simulink model "pos_control2"  (R2016b)
settings: Solver=ode3  StartTime=0.0  StopTime=50  FixedStep=0.0025  RelTol=1e-3
model workspace: external: MATLAB File /home/zhouhua/Clobotics/px4_simulink/px4_motor_order/pos_control_px4_order/para_pos.m (data not in the file)
values from neighbouring files (symbols this model uses):
  Ang_Pos_initial = [x0, y0, z0, phi0, theta0, psi0]    [para_pos.m]
  b = (middle_cruise_speed - c) / a    [get_vel_close.m]    (also in gradual.m = y_low - a * x_low; para_pos.m = 1.38089806e-06)
  compensation_gain = 1    [para_pos.m]
  d = 4.152245751114358e-08    (= 4.15224575111e-08)    [para_pos.m]
  dt = 0.0025    [para_pos.m]
  g = 9.8    [para_pos.m]
  Ix = 0.676603    [para_pos.m]
  Iy = 0.996394    [para_pos.m]
  Iz = 0.640393    [para_pos.m]
  L = 0.6    [para_pos.m]
  m = 10.3551    [para_pos.m]
  omiga1 = 0000    (= 0)    [para_pos.m]
  omiga2 = 0000    (= 0)    [para_pos.m]
  omiga3 = 0000    (= 0)    [para_pos.m]
  omiga4 = 0000    (= 0)    [para_pos.m]
  thrust_rpyt_low = [0,0,0,0,0,0]    [para_pos.m]
  thrust_rpyt_up = [1,1,1,1,1,1]    [para_pos.m]
  X1_PWM_MotorVel = -0.0023    [para_pos.m]
  X2_PWM_MotorVel = 13.6492    [para_pos.m]
  X3_PWM_MotorVel = -1.2185e+4    (= -12185)    [para_pos.m]
undefined symbols (not defined in the file or in its folder): bool_pos, control_mode, def, par, par_input, par_pos, position_setpoint
libraries: simulink x1
(part 1 of 2)
settings Model: Creator=root  LastModifiedBy=zhouhua
settings OptimizationCC: DefaultParameterBehavior=Inlined
settings DebuggingCC: ParameterTunabilityLossMsg=error
settings HardwareCC: ProdBitPerLong=64  ProdHWDeviceType=Intel->x86-64 (Linux 64)
settings RTWCC: SystemTargetFile=ert.tlc  TemplateMakefile=ert_default_tmf  Description=Embedded Coder  GenerateReport=on  IncludeHyperlinkInReport=on  LaunchReport=on  GenerateTraceInfo=on  GenerateTraceReport=on  GenerateTraceReportSl=on  GenerateTraceReportSf=on  GenerateTraceReportEml=on
settings CodeAppCC: ForceParamTrailComments=on  IgnoreCustomStorageClasses=off  OperatorAnnotations=on  SimulinkDataObjDesc=on  SFDataObjDesc=on  MATLABFcnDesc=on  InsertBlockDesc=on  MATLABSourceComments=on
settings ERTTargetCC: TargetLangStandard=C99 (ISO)  GenerateSampleERTMain=on  InlinedParameterPlacement=NonHierarchical  ERTCustomFileTemplate=example_file_process.tlc

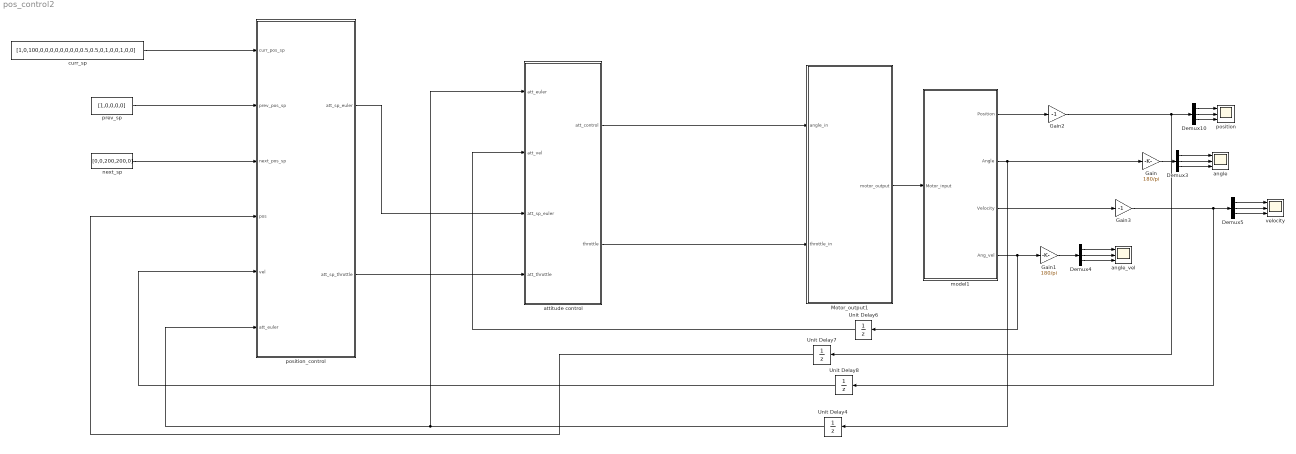
== system pos_control2 ==
  Demux{3..5,10} (4 alike) : Demux  Outputs=3
  Gain : Gain  Gain=180/pi
  Gain1 : Gain  Gain=180/pi
  Gain2 : Gain  Gain=-1
  Gain3 : Gain  Gain=-1
  Motor_output1 : Subsystem
  Unit Delay{4,6..8} (4 alike) : UnitDelay  InitialCondition=[0,0,0]  SampleTime=-1
  angle : Scope  NumInputPorts=3
  angle_vel : Scope  NumInputPorts=3
  attitude control : Subsystem
  curr_sp : Constant  Value=[1,0,100,0,0,0,0,0,0,0,0,0.5,0.5,0,1,0,0,1,0,0]
  model1 : Subsystem
  next_sp : Constant  Value=[0,0,200,200,0]
  position : Scope  NumInputPorts=3
  position_control : Subsystem
  prev_sp : Constant  Value=[1,0,0,0,0]
  velocity : Scope  NumInputPorts=3
  wires:
  Unit Delay4/1 -> position_control/6(att_euler), attitude control/1(att_euler)
  Unit Delay7/1 -> position_control/4(pos)
  Unit Delay8/1 -> position_control/5(vel)
  model1/2(Angle) -> Gain/1, Unit Delay4/1
  model1/4(Ang_vel) -> Gain1/1, Unit Delay6/1
  Gain2/1 -> Unit Delay7/1, Demux10/1
  model1/1(Position) -> Gain2/1
  Gain/1 -> Demux3/1
  Demux3/1 -> angle/1
  Demux3/2 -> angle/2
  Demux3/3 -> angle/3
  Demux4/1 -> angle_vel/1
  Demux4/2 -> angle_vel/2
  Demux4/3 -> angle_vel/3
  model1/3(Velocity) -> Gain3/1
  Demux5/1 -> velocity/1
  Demux5/2 -> velocity/2
  Demux5/3 -> velocity/3
  Gain1/1 -> Demux4/1
  Unit Delay6/1 -> attitude control/2(att_vel)
  Demux10/1 -> position/1
  Demux10/2 -> position/2
  Demux10/3 -> position/3
  Gain3/1 -> Demux5/1, Unit Delay8/1
  attitude control/1(att_control) -> Motor_output1/1(angle_in)
  attitude control/2(throttle) -> Motor_output1/2(throttle_in)
  position_control/1(att_sp_euler) -> attitude control/3(att_sp_euler)
  position_control/2(att_sp_throttle) -> attitude control/4(att_throttle)
  curr_sp/1 -> position_control/1(curr_pos_sp)
  prev_sp/1 -> position_control/2(prev_pos_sp)
  next_sp/1 -> position_control/3(next_pos_sp)
  Motor_output1/1(motor_output) -> model1/1(Motor_input)

== system pos_control2/Motor_output1 ==
  angle_in : Inport
  throttle_in : Inport  Port=2
  Display : Display
  output_armed_stabilizing : Subsystem
  output_to_motors : Subsystem
  motor_output : Outport
  wires:
  angle_in/1 -> Display/1, output_armed_stabilizing/1(In1)
  throttle_in/1 -> output_armed_stabilizing/2(In2)  "[0,1]"
  output_armed_stabilizing/1(thrust_rpyt_out) -> output_to_motors/1(thrust_in)
  output_to_motors/1(motor_ouput) -> motor_output/1

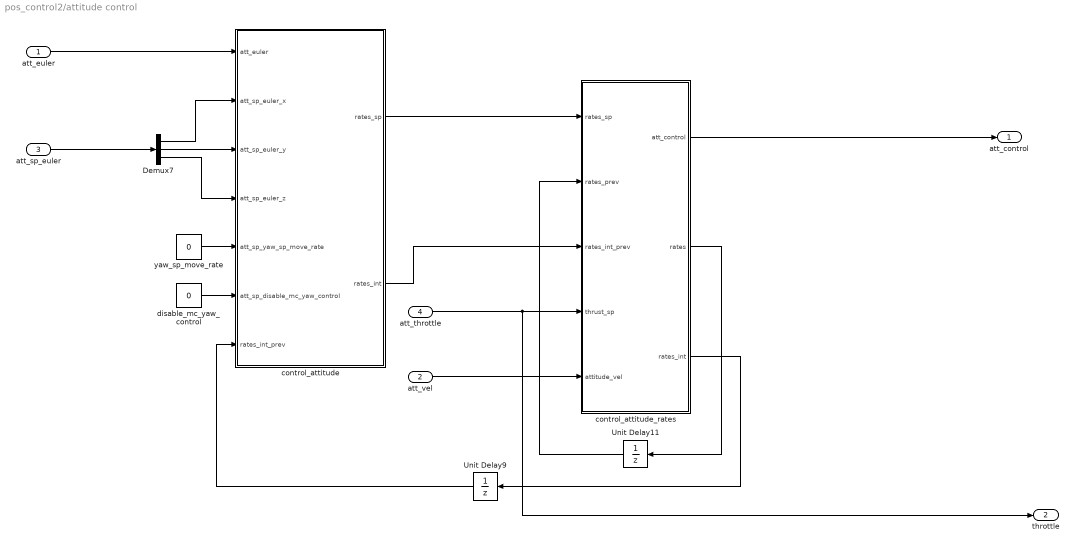
== system pos_control2/attitude control ==
  att_euler : Inport
  att_vel : Inport  Port=2
  att_sp_euler : Inport  Port=3
  att_throttle : Inport  Port=4
  Demux7 : Demux  Outputs=3
  Unit Delay11 : UnitDelay  InitialCondition=[0,0,0]  SampleTime=-1
  Unit Delay9 : UnitDelay  InitialCondition=[0,0,0]  SampleTime=-1
  control_attitude : MATLAB Function  TreatAsAtomicUnit=on
  control_attitude_rates : MATLAB Function  TreatAsAtomicUnit=on
  disable_mc_yaw_control : Constant  Value=0
  yaw_sp_move_rate : Constant  Value=0
  att_control : Outport
  throttle : Outport  Port=2
  wires:
  att_euler/1 -> control_attitude/1(att_euler)
  control_attitude_rates/3(rates_int) -> Unit Delay9/1
  control_attitude/2(rates_int) -> control_attitude_rates/3(rates_int_prev)
  control_attitude_rates/2(rates) -> Unit Delay11/1
  Unit Delay9/1 -> control_attitude/7(rates_int_prev)
  Unit Delay11/1 -> control_attitude_rates/2(rates_prev)
  yaw_sp_move_rate/1 -> control_attitude/5(att_sp_yaw_sp_move_rate)
  disable_mc_yaw_control/1 -> control_attitude/6(att_sp_disable_mc_yaw_control)
  control_attitude_rates/1(att_control) -> att_control/1
  control_attitude/1(rates_sp) -> control_attitude_rates/1(rates_sp)
  att_vel/1 -> control_attitude_rates/5(attitude_vel)
  Demux7/1 -> control_attitude/2(att_sp_euler_x)
  Demux7/2 -> control_attitude/3(att_sp_euler_y)
  Demux7/3 -> control_attitude/4(att_sp_euler_z)
  att_throttle/1 -> throttle/1, control_attitude_rates/4(thrust_sp)
  att_sp_euler/1 -> Demux7/1

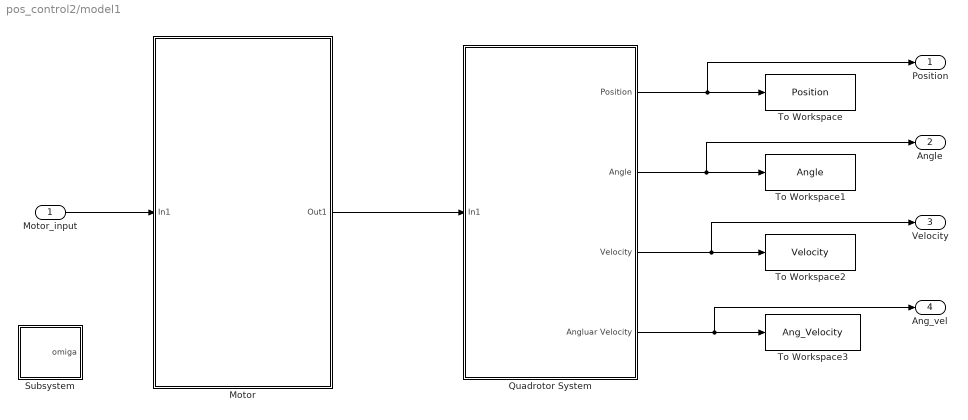
== system pos_control2/model1 ==
  Motor_input : Inport
  " Quadrotor System" : Subsystem
  Motor : Subsystem
  Subsystem : Subsystem
  To Workspace : ToWorkspace  VariableName=Position  SampleTime=-1
  To Workspace1 : ToWorkspace  VariableName=Angle  SampleTime=-1
  To Workspace2 : ToWorkspace  VariableName=Velocity  SampleTime=-1
  To Workspace3 : ToWorkspace  VariableName=Ang_Velocity  SampleTime=-1
  Position : Outport
  Angle : Outport  Port=2
  Velocity : Outport  Port=3
  Ang_vel : Outport  Port=4
  wires:
  Motor/1(Out1) -> " Quadrotor System"/1(In1)
  " Quadrotor System"/1(Position) -> Position/1, To Workspace/1
  " Quadrotor System"/3(Velocity) -> Velocity/1, To Workspace2/1
  " Quadrotor System"/4(Angluar Velocity) -> Ang_vel/1, To Workspace3/1
  Motor_input/1 -> Motor/1(In1)
  " Quadrotor System"/2(Angle) -> Angle/1, To Workspace1/1

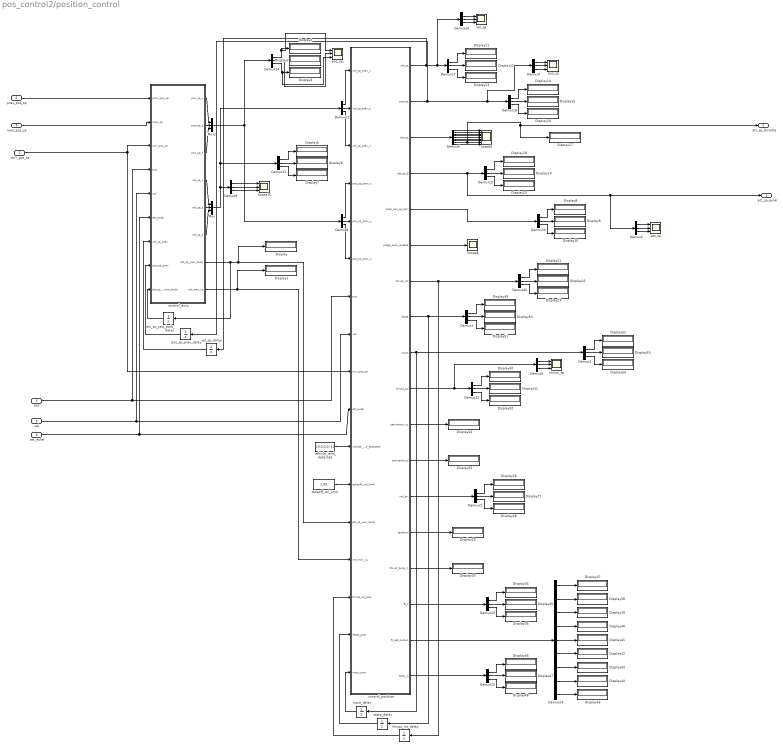
== system pos_control2/position_control ==
  curr_pos_sp : Inport
  prev_pos_sp : Inport  Port=2
  next_pos_sp : Inport  Port=3
  pos : Inport  Port=4
  vel : Inport  Port=5
  att_euler : Inport  Port=6
  Demux{1..5,8..10,12,14..23,25} (20 alike) : Demux  Outputs=3
  Demux24 : Demux  Outputs=9
  Demux6 : Demux  Outputs=9
  Display{,1..54} (55 alike) : Display
  Mux : Mux  Inputs=3
  Mux1 : Mux  Inputs=3
  Scope10 : Scope  NumInputPorts=3
  Scope5 : Scope  NumInputPorts=9
  Scope6 : Scope
  att_sp : Scope  NumInputPorts=3
  att_sp_yaw_body_delay : UnitDelay  InitialCondition=[0]  SampleTime=-1
  control_auto : MATLAB Function  TreatAsAtomicUnit=on
  control_position : MATLAB Function  TreatAsAtomicUnit=on
  input_delay : UnitDelay  InitialCondition=[0,0,0]  SampleTime=-1
  pos_sp : Scope  NumInputPorts=3
  "pos_sp_ " : Scope  NumInputPorts=3
  pos_sp_prev_delay : UnitDelay  InitialCondition=[0]  SampleTime=-1
  state_delay : UnitDelay  InitialCondition=[0,0,0]  SampleTime=-1
  takeoff_vel_limit : Constant  Value=1.53
  thrust_int_delay : UnitDelay  InitialCondition=[0,0,0]  SampleTime=-1
  thrust_sp : Scope  NumInputPorts=3
  vehicle_land_detected : Constant  Value=[0,0,0,0,-1]
  vel_sp : Scope  NumInputPorts=3
  vel_sp_delay : UnitDelay  InitialCondition=[0]  SampleTime=-1
  att_sp_euler : Outport
  att_sp_throttle : Outport  Port=2
  wires:
  control_auto/7(att_sp_yaw_body) -> att_sp_yaw_body_delay/1, Display/1, control_position/13(att_sp_yaw_body)
  control_auto/8(vel_max_xy) -> Display1/1, control_position/14(vel_max_xy)
  takeoff_vel_limit/1 -> control_position/12(takeoff_vel_limit)
  vehicle_land_detected/1 -> control_position/11(vehicle_land_detected)
  next_pos_sp/1 -> control_auto/2(next_sp)
  prev_pos_sp/1 -> control_auto/1(prev_pos_sp)
  curr_pos_sp/1 -> control_auto/3(curr_pos_sp), control_position/9(curr_pos_sp)
  Demux6/1 -> Scope5/1
  Demux6/2 -> Scope5/2
  Demux6/3 -> Scope5/3
  control_position/3(att_sp) -> Demux6/1
  Demux6/4 -> Scope5/4
  Demux6/5 -> Scope5/5
  Demux6/6 -> Scope5/6
  Demux6/7 -> Scope5/7
  Demux6/9 -> Scope5/9
  control_position/5(local_pos_sp_acc) -> Demux16/1
  control_position/6(judge_auto_enable) -> Scope6/1
  Demux8/1 -> control_position/4(pos_sp_prev_x)
  Demux8/2 -> control_position/5(pos_sp_prev_y)
  Demux8/3 -> control_position/6(pos_sp_prev_z)
  Demux9/1 -> Scope10/1
  Demux9/2 -> Scope10/2
  Demux9/3 -> Scope10/3
  Mux1/1 -> Demux8/1, Demux14/1
  Demux12/1 -> control_position/1(vel_sp_prev_x)
  Demux12/2 -> control_position/2(vel_sp_prev_y)
  Demux12/3 -> control_position/3(vel_sp_prev_z)
  Demux14/2 -> "pos_sp_ "/2, Display3/1
  Demux14/3 -> "pos_sp_ "/3, Display4/1
  Demux14/1 -> "pos_sp_ "/1, Display2/1
  Mux/1 -> Demux12/1, Demux15/1, Demux9/1
  Demux15/2 -> Display6/1
  Demux15/3 -> Display7/1
  Demux15/1 -> Display5/1
  att_euler/1 -> control_position/10(att_euler), control_auto/6(att_euler)
  pos/1 -> control_position/7(pos), control_auto/4(pos)
  vel/1 -> control_position/8(vel), control_auto/5(vel)
  Demux16/2 -> Display9/1
  Demux16/3 -> Display10/1
  Demux16/1 -> Display8/1
  Demux17/2 -> Display12/1
  Demux17/3 -> Display13/1
  Demux17/1 -> Display11/1
  Demux18/2 -> Display15/1
  Demux18/3 -> Display16/1
  Demux18/1 -> Display14/1
  Demux19/2 -> Display19/1
  Demux19/3 -> Display20/1
  Demux19/1 -> Display18/1
  control_position/7(thrust_int) -> thrust_int_delay/1, Demux20/1
  Demux20/2 -> Display22/1
  Demux20/3 -> Display23/1
  Demux20/1 -> Display21/1
  control_position/11(saturation_xy) -> Display24/1
  control_position/12(saturation_z) -> Display25/1
  control_position/13(vel_err) -> Demux21/1
  Demux21/2 -> Display27/1
  Demux21/3 -> Display28/1
  Demux21/1 -> Display26/1
  control_position/14(testbool) -> Display29/1
  Demux22/2 -> Display31/1
  Demux22/3 -> Display32/1
  Demux22/1 -> Display30/1
  control_position/15(thrust_body_z) -> Display33/1
  Demux23/2 -> Display35/1
  Demux23/3 -> Display36/1
  Demux23/1 -> Display34/1
  control_position/16(R_z) -> Demux23/1
  Demux24/1 -> Display37/1
  Demux24/2 -> Display38/1
  Demux24/3 -> Display39/1
  Demux24/4 -> Display40/1
  Demux24/5 -> Display41/1
  Demux24/6 -> Display42/1
  Demux24/7 -> Display43/1
  Demux24/8 -> Display44/1
  Demux24/9 -> Display45/1
  control_position/17(R_set_output) -> Demux24/1
  Demux25/2 -> Display47/1
  Demux25/3 -> Display48/1
  Demux25/1 -> Display46/1
  control_position/18(body_z) -> Demux25/1
  state_delay/1 -> control_position/16(State_prev)
  Demux1/2 -> Display50/1
  Demux1/3 -> Display51/1
  Demux1/1 -> Display49/1
  control_position/8(State) -> state_delay/1, Demux1/1
  input_delay/1 -> control_position/17(input_prev)
  Demux2/2 -> Display53/1
  Demux2/3 -> Display54/1
  Demux2/1 -> Display52/1
  control_position/9(input) -> input_delay/1, Demux2/1
  thrust_int_delay/1 -> control_position/15(thrust_int_prev)
  att_sp_yaw_body_delay/1 -> control_auto/9(att_sp_prev_yaw_body)
  vel_sp_delay/1 -> control_auto/7(vel_sp_prev)
  Demux6/8 -> Scope5/8, Display17/1, att_sp_throttle/1
  control_auto/5(vel_sp_y) -> Mux/2
  control_auto/4(vel_sp_x) -> Mux/1
  control_auto/6(vel_sp_z) -> Mux/3
  control_auto/2(pos_sp_y) -> Mux1/2
  control_auto/3(pos_sp_z) -> Mux1/3
  control_auto/1(pos_sp_x) -> Mux1/1
  control_position/1(vel_sp) -> vel_sp_delay/1, Demux10/1, Demux17/1
  Demux10/1 -> vel_sp/1
  Demux10/2 -> vel_sp/2
  Demux10/3 -> vel_sp/3
  control_position/2(pos_sp) -> pos_sp_prev_delay/1, Demux3/1, Demux18/1
  Demux3/1 -> pos_sp/1
  Demux3/2 -> pos_sp/2
  Demux3/3 -> pos_sp/3
  control_position/4(att_sp_3) -> Demux4/1, att_sp_euler/1, Demux19/1
  Demux4/1 -> att_sp/1
  Demux4/2 -> att_sp/2
  Demux4/3 -> att_sp/3
  control_position/10(thrust_sp) -> Demux5/1, Demux22/1
  Demux5/1 -> thrust_sp/1
  Demux5/2 -> thrust_sp/2
  Demux5/3 -> thrust_sp/3
  pos_sp_prev_delay/1 -> control_auto/8(pos_sp_prev)

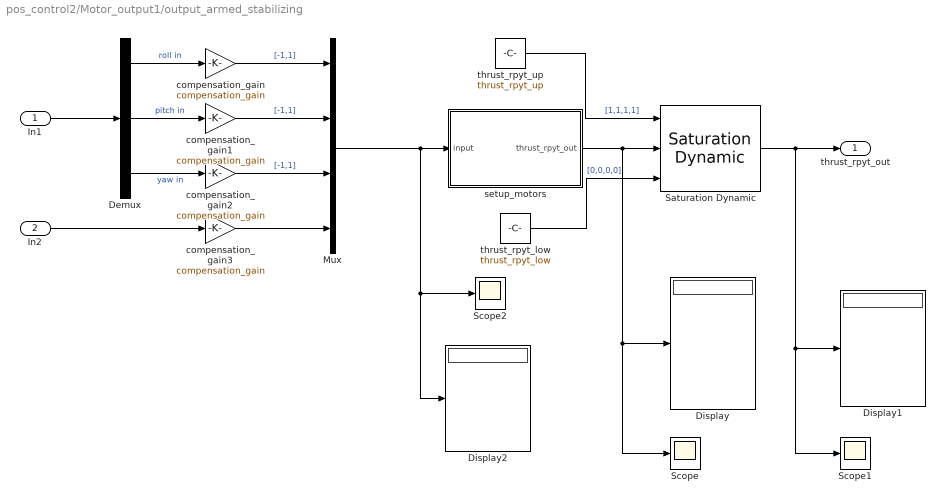
== system pos_control2/Motor_output1/output_armed_stabilizing ==
  In1 : Inport
  In2 : Inport  Port=2
  Demux : Demux  Outputs=3
  Display : Display
  Display1 : Display
  Display2 : Display
  Mux : Mux
  Saturation Dynamic : simulink/Discontinuities/Saturation Dynamic  OutMin=[]  OutMax=[]  OutDataTypeStr=Inherit: Same as second input  OutDataType=fixdt(1, 16)  OutScaling=2^-10  DoSatur=off
  Scope : Scope
  Scope1 : Scope
  Scope2 : Scope
  compensation_gain{,1..3} (4 alike) : Gain  Gain=compensation_gain
  setup_motors : MATLAB Function  TreatAsAtomicUnit=on
  thrust_rpyt_low : Constant  Value=thrust_rpyt_low
  thrust_rpyt_up : Constant  Value=thrust_rpyt_up
  thrust_rpyt_out : Outport
  wires:
  thrust_rpyt_up/1 -> Saturation Dynamic/1  "[1,1,1,1]"
  setup_motors/1(thrust_rpyt_out) -> Scope/1, Display/1, Saturation Dynamic/2
  In1/1 -> Demux/1
  compensation_gain1/1 -> Mux/2  "[-1,1]"
  compensation_gain/1 -> Mux/1  "[-1,1]"
  compensation_gain2/1 -> Mux/3  "[-1,1]"
  compensation_gain3/1 -> Mux/4
  In2/1 -> compensation_gain3/1
  Demux/1 -> compensation_gain/1  "roll in"
  Demux/3 -> compensation_gain2/1  "yaw in"
  Demux/2 -> compensation_gain1/1  "pitch in"
  Saturation Dynamic/1 -> Scope1/1, Display1/1, thrust_rpyt_out/1
  thrust_rpyt_low/1 -> Saturation Dynamic/3  "[0,0,0,0]"
  Mux/1 -> setup_motors/1(input), Display2/1, Scope2/1

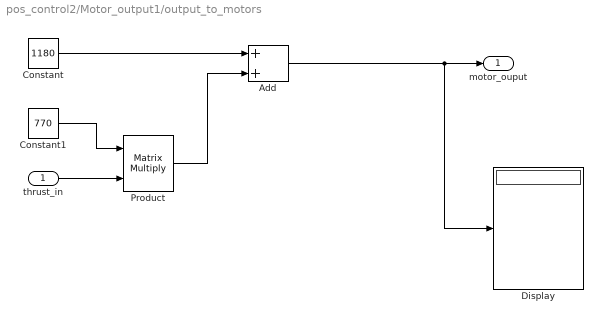
== system pos_control2/Motor_output1/output_to_motors ==
  thrust_in : Inport
  Add : Sum
  Constant : Constant  Value=1180
  Constant1 : Constant  Value=770
  Display : Display
  Product : Product  Multiplication=Matrix(*)
  motor_ouput : Outport
  wires:
  thrust_in/1 -> Product/2
  Constant1/1 -> Product/1
  Constant/1 -> Add/1
  Product/1 -> Add/2
  Add/1 -> Display/1, motor_ouput/1

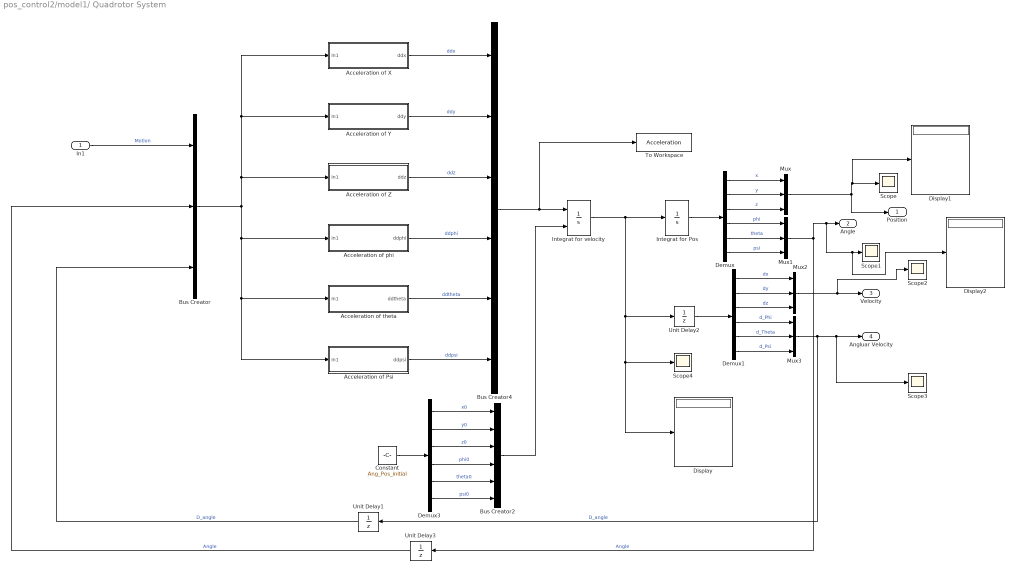
== system pos_control2/model1/ Quadrotor System ==
  In1 : Inport
  Acceleration of Psi : Subsystem
  Acceleration of X : Subsystem
  Acceleration of Y : Subsystem
  Acceleration of Z : Subsystem
  Acceleration of phi : Subsystem
  Acceleration of theta : Subsystem
  Bus Creator : BusCreator  Inputs=3
  Bus Creator2 : BusCreator  Inputs=6
  Bus Creator4 : BusCreator  Inputs=6
  Constant : Constant  Value=Ang_Pos_initial
  Demux : Demux  Outputs=6
  Demux1 : Demux  Outputs=6
  Demux3 : Demux  Outputs=6
  Display : Display
  Display1 : Display
  Display2 : Display
  Integrat for Pos : Integrator  InitialCondition=zeros(6,1)
  Integrat for velocity : Integrator  InitialConditionSource=external  InitialCondition=zeros(6,1)
  Mux{,1..3} (4 alike) : Mux  Inputs=3
  Scope{,1..4} (5 alike) : Scope
  To Workspace : ToWorkspace  VariableName=Acceleration  SaveFormat=Structure  SampleTime=-1
  Unit Delay1 : UnitDelay  InitialCondition=zeros(3,1)  SampleTime=-1
  Unit Delay2 : UnitDelay  InitialCondition=zeros(6,1)  SampleTime=-1
  Unit Delay3 : UnitDelay  InitialCondition=zeros(3,1)  SampleTime=-1
  Position : Outport
  Angle : Outport  Port=2
  Velocity : Outport  Port=3
  Angluar Velocity : Outport  Port=4
  wires:
  In1/1 -> Bus Creator/1  "Motion"
  Bus Creator/1 -> Acceleration of Psi/1(In1), Acceleration of theta/1(In1), Acceleration of phi/1(In1), Acceleration of Y/1(In1), Acceleration of X/1(In1), Acceleration of Z/1(In1)
  Acceleration of X/1(ddx) -> Bus Creator4/1  "ddx"
  Acceleration of Y/1(ddy) -> Bus Creator4/2  "ddy"
  Acceleration of Z/1(ddz) -> Bus Creator4/3  "ddz"
  Acceleration of phi/1(ddphi) -> Bus Creator4/4  "ddphi"
  Acceleration of theta/1(ddtheta) -> Bus Creator4/5  "ddtheta"
  Acceleration of Psi/1(ddpsi) -> Bus Creator4/6  "ddpsi"
  Bus Creator4/1 -> To Workspace/1, Integrat for velocity/1
  Integrat for velocity/1 -> Integrat for Pos/1, Display/1, Scope4/1, Unit Delay2/1
  Demux/1 -> Mux/1  "x"
  Demux/2 -> Mux/2  "y"
  Demux/3 -> Mux/3  "z"
  Demux/4 -> Mux1/1  "phi"
  Demux/5 -> Mux1/2  "theta"
  Demux/6 -> Mux1/3  "psi"
  Demux1/1 -> Mux2/1  "dx"
  Demux1/2 -> Mux2/2  "dy"
  Demux1/3 -> Mux2/3  "dz"
  Demux1/4 -> Mux3/1  "d_Phi"
  Demux1/5 -> Mux3/2  "d_Theta"
  Demux1/6 -> Mux3/3  "d_Psi"
  Mux3/1 -> Unit Delay1/1, Scope3/1, Angluar Velocity/1  "D_angle"
  Mux2/1 -> Scope2/1, Velocity/1
  Constant/1 -> Demux3/1
  Demux3/1 -> Bus Creator2/1  "x0"
  Demux3/2 -> Bus Creator2/2  "y0"
  Demux3/3 -> Bus Creator2/3  "z0"
  Demux3/4 -> Bus Creator2/4  "phi0"
  Demux3/5 -> Bus Creator2/5  "theta0"
  Demux3/6 -> Bus Creator2/6  "psi0"
  Bus Creator2/1 -> Integrat for velocity/2
  Unit Delay2/1 -> Demux1/1
  Integrat for Pos/1 -> Demux/1
  Mux1/1 -> Display2/1, Scope1/1, Angle/1, Unit Delay3/1  "Angle"
  Mux/1 -> Position/1, Display1/1, Scope/1
  Unit Delay1/1 -> Bus Creator/3  "D_angle"
  Unit Delay3/1 -> Bus Creator/2  "Angle"

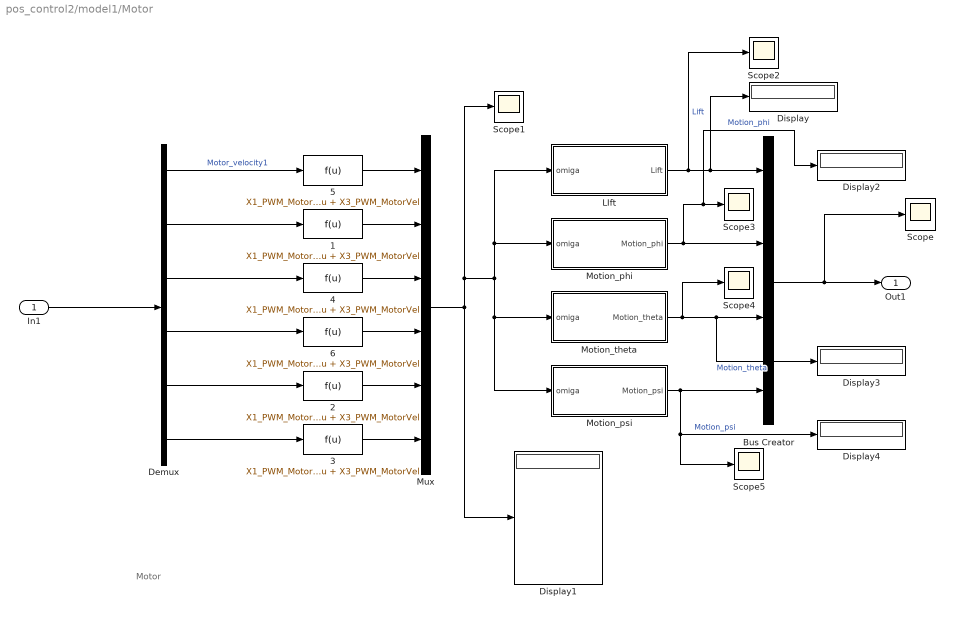
== system pos_control2/model1/Motor ==
  note: Motor
  In1 : Inport
  {1..6} (6 alike) : Fcn  Expr=X1_PWM_MotorVel * u^2 + X2_PWM_MotorVel * u + X3_PWM_MotorVel
  Bus Creator : BusCreator  Inputs=4
  Demux : Demux  Outputs=6
  Display{,1..4} (5 alike) : Display
  LIft : Subsystem
  Motion_phi : Subsystem
  Motion_psi : Subsystem
  Motion_theta : Subsystem
  Mux : Mux  Inputs=6
  Scope{,1..5} (6 alike) : Scope
  Out1 : Outport
  wires:
  LIft/1(Lift) -> Scope2/1, Display/1, Bus Creator/1  "Lift"
  Motion_phi/1(Motion_phi) -> Bus Creator/2, Display2/1, Scope3/1  "Motion_phi"
  Motion_theta/1(Motion_theta) -> Display3/1, Bus Creator/3, Scope4/1  "Motion_theta"
  Motion_psi/1(Motion_psi) -> Display4/1, Scope5/1, Bus Creator/4  "Motion_psi"
  Mux/1 -> Scope1/1, Motion_psi/1(omiga), Motion_theta/1(omiga), Motion_phi/1(omiga), LIft/1(omiga), Display1/1
  Demux/1 -> 5/1  "Motor_velocity1"
  Demux/2 -> 1/1
  Demux/3 -> 4/1
  Demux/4 -> 6/1
  Bus Creator/1 -> Scope/1, Out1/1
  In1/1 -> Demux/1
  5/1 -> Mux/1
  6/1 -> Mux/4
  4/1 -> Mux/3
  1/1 -> Mux/2
  Demux/5 -> 2/1
  2/1 -> Mux/5
  Demux/6 -> 3/1
  3/1 -> Mux/6

== system pos_control2/model1/Subsystem ==
  Bus Creator : BusCreator  Inputs=4
  Constant : Constant  Value=omiga1
  Constant2 : Constant  Value=omiga2
  Constant3 : Constant  Value=omiga3
  Constant4 : Constant  Value=omiga4
  omiga : Outport
  wires:
  Constant/1 -> Bus Creator/1  "omiga1"
  Constant2/1 -> Bus Creator/2  "omiga2"
  Constant3/1 -> Bus Creator/3  "omiga3"
  Constant4/1 -> Bus Creator/4  "omiga4"
  Bus Creator/1 -> omiga/1

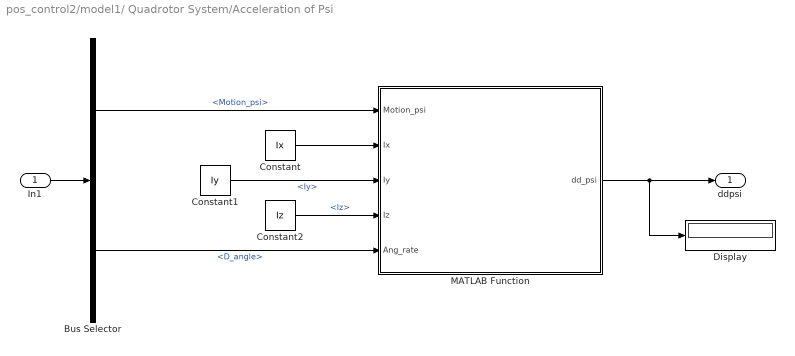
== system pos_control2/model1/ Quadrotor System/Acceleration of Psi ==
  In1 : Inport
  Bus Selector : BusSelector  OutputSignals=Motion.Motion_psi,D_angle
  Constant : Constant  Value=Ix
  Constant1 : Constant  Value=Iy
  Constant2 : Constant  Value=Iz
  Display : Display
  MATLAB Function : MATLAB Function  TreatAsAtomicUnit=on
  ddpsi : Outport
  wires:
  MATLAB Function/1(dd_psi) -> Display/1, ddpsi/1
  In1/1 -> Bus Selector/1
  Bus Selector/1 -> MATLAB Function/1(Motion_psi)  "<Motion_psi>"
  Constant1/1 -> MATLAB Function/3(Iy)  "<Iy>"
  Constant2/1 -> MATLAB Function/4(Iz)  "<Iz>"
  Bus Selector/2 -> MATLAB Function/5(Ang_rate)  "<D_angle>"
  Constant/1 -> MATLAB Function/2(Ix)

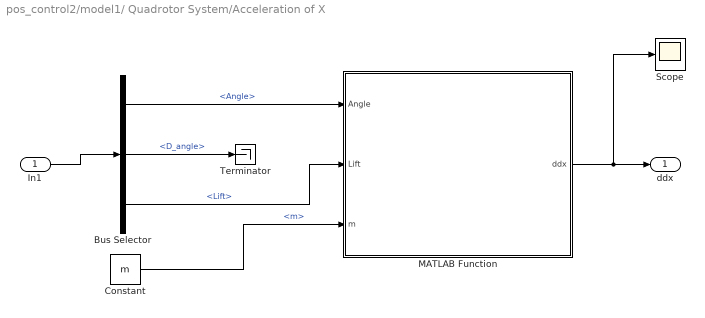
== system pos_control2/model1/ Quadrotor System/Acceleration of X ==
  In1 : Inport
  Bus Selector : BusSelector  OutputSignals=Angle,D_angle,Motion.Lift
  Constant : Constant  Value=m
  MATLAB Function : MATLAB Function  TreatAsAtomicUnit=on
  Scope : Scope
  Terminator : Terminator
  ddx : Outport
  wires:
  In1/1 -> Bus Selector/1
  Bus Selector/1 -> MATLAB Function/1(Angle)  "<Angle>"
  Bus Selector/2 -> Terminator/1  "<D_angle>"
  Bus Selector/3 -> MATLAB Function/2(Lift)  "<Lift>"
  MATLAB Function/1(ddx) -> Scope/1, ddx/1
  Constant/1 -> MATLAB Function/3(m)  "<m>"

== system pos_control2/model1/ Quadrotor System/Acceleration of Y ==
  In1 : Inport
  Bus Selector : BusSelector  OutputSignals=Angle,Motion.Lift
  Constant : Constant  Value=m
  Display : Display
  MATLAB Function : MATLAB Function  TreatAsAtomicUnit=on
  Scope : Scope
  ddy : Outport
  wires:
  In1/1 -> Bus Selector/1
  Bus Selector/1 -> MATLAB Function/1(Angle)  "<Angle>"
  Bus Selector/2 -> MATLAB Function/2(List)  "<Lift>"
  MATLAB Function/1(ddy) -> Display/1, Scope/1, ddy/1
  Constant/1 -> MATLAB Function/3(m)  "<m>"

== system pos_control2/model1/ Quadrotor System/Acceleration of Z ==
  In1 : Inport
  Bus Selector : BusSelector  OutputSignals=Angle,Motion.Lift
  Constant : Constant  Value=m
  Constant1 : Constant  Value=g
  MATLAB Function : MATLAB Function  TreatAsAtomicUnit=on
  Scope4 : Scope
  ddz : Outport
  wires:
  In1/1 -> Bus Selector/1
  Bus Selector/1 -> MATLAB Function/1(Angle)  "<Angle>"
  Bus Selector/2 -> MATLAB Function/2(List)  "<Lift>"
  MATLAB Function/1(ddz) -> Scope4/1, ddz/1
  Constant/1 -> MATLAB Function/3(m)  "<m>"
  Constant1/1 -> MATLAB Function/4(g)

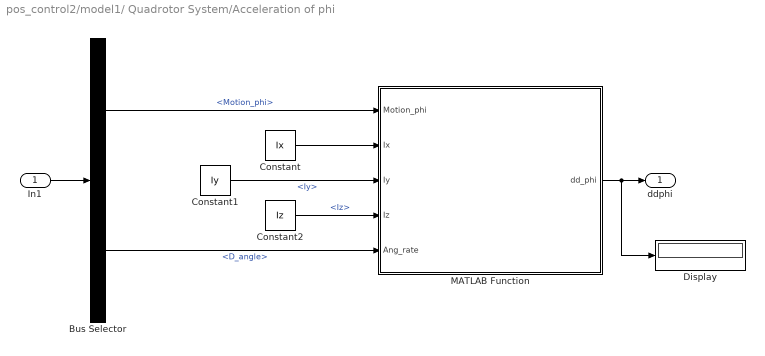
== system pos_control2/model1/ Quadrotor System/Acceleration of phi ==
  In1 : Inport
  Bus Selector : BusSelector  OutputSignals=Motion.Motion_phi,D_angle
  Constant : Constant  Value=Ix
  Constant1 : Constant  Value=Iy
  Constant2 : Constant  Value=Iz
  Display : Display
  MATLAB Function : MATLAB Function  TreatAsAtomicUnit=on
  ddphi : Outport
  wires:
  In1/1 -> Bus Selector/1
  Bus Selector/1 -> MATLAB Function/1(Motion_phi)  "<Motion_phi>"
  MATLAB Function/1(dd_phi) -> Display/1, ddphi/1
  Constant1/1 -> MATLAB Function/3(Iy)  "<Iy>"
  Constant2/1 -> MATLAB Function/4(Iz)  "<Iz>"
  Bus Selector/2 -> MATLAB Function/5(Ang_rate)  "<D_angle>"
  Constant/1 -> MATLAB Function/2(Ix)

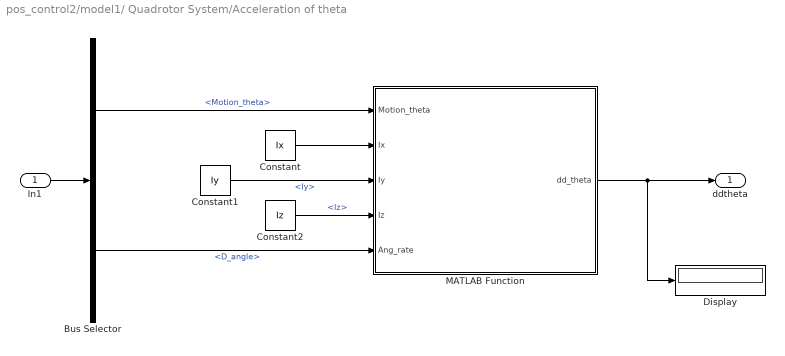
== system pos_control2/model1/ Quadrotor System/Acceleration of theta ==
  In1 : Inport
  Bus Selector : BusSelector  OutputSignals=Motion.Motion_theta,D_angle
  Constant : Constant  Value=Ix
  Constant1 : Constant  Value=Iy
  Constant2 : Constant  Value=Iz
  Display : Display
  MATLAB Function : MATLAB Function  TreatAsAtomicUnit=on
  ddtheta : Outport
  wires:
  In1/1 -> Bus Selector/1
  Bus Selector/1 -> MATLAB Function/1(Motion_theta)  "<Motion_theta>"
  Constant1/1 -> MATLAB Function/3(Iy)  "<Iy>"
  Constant2/1 -> MATLAB Function/4(Iz)  "<Iz>"
  Bus Selector/2 -> MATLAB Function/5(Ang_rate)  "<D_angle>"
  Constant/1 -> MATLAB Function/2(Ix)
  MATLAB Function/1(dd_theta) -> Display/1, ddtheta/1

== system pos_control2/model1/Motor/LIft ==
  omiga : Inport
  Display : Display
  Display1 : Display
  Fcn : Fcn  Expr=b * (u(1)^2 + u(2)^2 + u(3)^2 + u(4)^2 + u(5)^2 + u(6)^2)
  Lift : Outport
  wires:
  Fcn/1 -> Display1/1, Lift/1
  omiga/1 -> Display/1, Fcn/1

== system pos_control2/model1/Motor/Motion_phi ==
  omiga : Inport
  Display : Display
  Display1 : Display
  Fcn : Fcn  Expr=L * b * (-0.5*u(1)^2 -u(4)^2 - 0.5*u(5)^2 + 0.5*u(2)^2 + u(3)^2 + 0.5*u(6)^2 )
  Motion_phi : Outport
  wires:
  omiga/1 -> Display/1, Fcn/1
  Fcn/1 -> Display1/1, Motion_phi/1

== system pos_control2/model1/Motor/Motion_psi ==
  omiga : Inport
  Display : Display
  Display1 : Display
  Fcn : Fcn  Expr=d * (u(5)^2 + u(4)^2 - u(1)^2 - u(6)^2 +u(2)^2 -u(3)^2)
  Motion_psi : Outport
  wires:
  Fcn/1 -> Display1/1, Motion_psi/1
  omiga/1 -> Display/1, Fcn/1

== system pos_control2/model1/Motor/Motion_theta ==
  omiga : Inport
  Fcn : Fcn  Expr=sqrt(3)/2 * L * b * (u(5)^2 - u(4)^2 - u(6)^2 + u(3)^2)
  Motion_theta : Outport
  wires:
  Fcn/1 -> Motion_theta/1
  omiga/1 -> Fcn/1

== matlab function pos_control2/Motor_output1/output_armed_stabilizing/setup_motors ==
  data: thrust_rpyt_out output; input input
function thrust_rpyt_out = fcn(input)
thrust_rpyt_out = zeros(6,1);
motor_num = zeros(6,1);roll_factor_in_degrees = zeros(6,1); yaw_factor = zeros(6,1); roll_factor = zeros(6,1);pitch_factor = zeros(6,1);throttle_factor = zeros(6,1);
matrix_px4 = zeros(6,4);
% X frame set-up
motor_num(5) = 1; roll_factor_in_degrees(1) = pi / 6 ;      yaw_factor(1)= 1;  roll_factor(1) = -1/2; pitch_factor(1) = sqrt(3)/2;   throttle_factor(1) = 1;
motor_num(1) = 2; roll_factor_in_degrees(2) = pi / 2;       yaw_factor(2)= -1; roll_factor(2) = -1;   pitch_factor(2) = 0;           throttle_factor(2) = 1;
motor_num(4) = 3; roll_factor_in_degrees(3) =  5 * pi / 6;  yaw_factor(3)= 1;  roll_factor(3) = -1/2; pitch_factor(3) = -sqrt(3)/2;  throttle_factor(3) = 1;
motor_num(6) = 4; roll_factor_in_degrees(4) = -5 * pi / 6;  yaw_factor(4)= -1; roll_factor(4) = 1/2;  pitch_factor(4) = -sqrt(3)/2;  throttle_factor(4) = 1;
motor_num(2) = 5; roll_factor_in_degrees(5) = - pi / 2;     yaw_factor(5)= 1;  roll_factor(5) = 1;    pitch_factor(5) = 0;           throttle_factor(5) = 1;
motor_num(3) = 6; roll_factor_in_degrees(6) = - pi / 6;     yaw_factor(6)= -1; roll_factor(6) = 1/2;  pitch_factor(6) = sqrt(3)/2;   throttle_factor(6) = 1;

matrix = [ roll_factor(1), pitch_factor(1), yaw_factor(1), throttle_factor(1);
           roll_factor(2), pitch_factor(2), yaw_factor(2), throttle_factor(2);
           roll_factor(3), pitch_factor(3), yaw_factor(3), throttle_factor(3);
           roll_factor(4), pitch_factor(4), yaw_factor(4), throttle_factor(4);
           roll_factor(5), pitch_factor(5), yaw_factor(5), throttle_factor(5);
           roll_factor(6), pitch_factor(6), yaw_factor(6), throttle_factor(6)];
       matrix_px4(5,:) = matrix(1,:);
       matrix_px4(1,:) = matrix(2,:);
       matrix_px4(4,:) = matrix(3,:);
       matrix_px4(6,:) = matrix(4,:);
       matrix_px4(2,:) = matrix(5,:);
       matrix_px4(3,:) = matrix(6,:);
thrust_rpyt_out = matrix_px4 * input;

== matlab function pos_control2/model1/ Quadrotor System/Acceleration of Psi/MATLAB Function ==
  data: Motion_psi input; dd_psi output; Ix input; Iy input; Iz input; Ang_rate input
function dd_psi = fcn(Motion_psi, Ix, Iy, Iz, Ang_rate)
D_theta = Ang_rate(2); D_phi = Ang_rate(1);
dd_psi = D_theta * D_phi * (Ix - Iy) / Iz + Motion_psi / Iz;

== matlab function pos_control2/attitude control/control_attitude ==
  data: att_euler input; att_sp_euler_x input; att_sp_euler_y input; att_sp_euler_z input; rates_sp output; rates_int output; att_sp_yaw_sp_move_rate input; att_sp_disable_mc_yaw_control input; rates_int_prev input; par parameter; control_mode parameter
function [rates_sp,rates_int] = control_attitude(att_euler,att_sp_euler_x,att_sp_euler_y,att_sp_euler_z,att_sp_yaw_sp_move_rate,att_sp_disable_mc_yaw_control,rates_int_prev,par, control_mode)
%construct attitude setpoint rotation matrix
%get current rotation matrix from control state quaternions
rates_int = rates_int_prev;
I = diag([1,1,1]);
att_sp_euler = [att_sp_euler_x,att_sp_euler_y,att_sp_euler_z]';
R_sp = euler_to_dcm(att_sp_euler);
R = euler_to_dcm(att_euler);
%R = q_to_dcm(v_att_q);
%try to move thrust vector shortest way, because yaw response is slower than roll/pitch
R_z = [R(1,3),R(2,3),R(3,3)]';
R_sp_z = [R_sp(1,3),R_sp(2,3),R_sp(3,3)]';

%axis and sin(angle) of desired rotation (indexes: 0=pitch, 1=roll, 2=yaw).
%This is for roll/pitch only (tilt), e_R(2) is 0
e_R = R'* cross(R_z,R_sp_z);

%calculate angle error
e_R_z_sin = norm(e_R);
e_R_z_cos = dot(R_z,R_sp_z);

%calculate rotation matrix after roll/pitch only rotation
R_rp = zeros(3);

if e_R_z_sin > 0.0
    %get axis-angle representation
    e_R_z_angle = atan(e_R_z_sin/e_R_z_cos);
    e_R_z_axis = e_R/e_R_z_sin;
    
    e_R = e_R_z_axis*e_R_z_angle;
    
    %cross product matrix for e_R_axis
    e_R_cp = zeros(3);
	e_R_cp(1, 2) = -e_R_z_axis(3);
	e_R_cp(1, 3) = e_R_z_axis(2);
	e_R_cp(2, 1) = e_R_z_axis(3);
	e_R_cp(2, 3) = -e_R_z_axis(1);
	e_R_cp(3, 1) = -e_R_z_axis(2);
	e_R_cp(3, 2) = e_R_z_axis(1);
    %rotation matrix for roll/pitch only rotation
    R_rp = R * (I + e_R_cp * e_R_z_sin + e_R_cp * e_R_cp * (1.0 - e_R_z_cos));
else
    %zero roll/pitch rotation 
    R_rp = R;
end

% R_rp and R_sp have the same Z axis, calculate yaw error 
R_sp_x = [R_sp(1, 1), R_sp(2, 1), R_sp(3, 1)]';
R_rp_x = [R_rp(1, 1), R_rp(2, 1), R_rp(3, 1)]';
    
%  calculate the weight for yaw control
%  Make the weight depend on the tilt angle error: the higher the error of roll and/or pitch, the lower
%  the weight that we use to control the yaw. This gives precedence to roll & pitch correction.
%  The weight is 1 if there is no tilt error.
yaw_w = e_R_z_cos*e_R_z_cos;

e_R(3) = atan(dot(cross(R_rp_x,R_sp_x),R_sp_z)/dot(R_rp_x,R_sp_x)) * yaw_w;
if e_R_z_cos<0.0
    q_error = dcm_to_q(R'*R_sp);
    if q_error >= 0.0
        e_R_d = [q_error(2),q_error(3),q_error(4)]'*2;
    else
        e_R_d = [-q_error(2),-q_error(3),-q_error(4)]'*2;
    end
    % use fusion of Z axis based rotation and direct rotation
    direct_w = e_R_z_cos * e_R_z_cos * yaw_w;
    e_R = e_R * (1.0 - direct_w) + e_R_d * direct_w;
end

% calculate angular rates setpoint
rates_sp = [par.att_p(1)*e_R(1),par.att_p(2)*e_R(2),par.att_p(3)*e_R(3)]';
% Feed forward the yaw setpoint rate. We need to transform the yaw from world into body frame.
% The following is a simplification of:
yaw_feedforward_rate = [R(3, 1), R(3, 2), R(3, 3)]';
yaw_feedforward_rate = yaw_feedforward_rate * att_sp_yaw_sp_move_rate * par.yaw_ff;

yaw_feedforward_rate(3) = yaw_feedforward_rate(3) * yaw_w;
rates_sp = rates_sp + yaw_feedforward_rate;

% limit rates
for i = 1:2
    if (control_mode.flag_control_velocity_enabled || control_mode.flag_control_auto_enabled) && ~control_mode.flag_control_manual_enabled
        rates_sp(i) = constrain(rates_sp(i), -par.auto_rate_max(i), par.auto_rate_max(i));
    else
        rates_sp(i) = constrain(rates_sp(i), -par.mc_rate_max(i), par.mc_rate_max(i));
    end
end
        
if (control_mode.flag_control_velocity_enabled || control_mode.flag_control_auto_enabled) && att_sp_disable_mc_yaw_control == true && ~control_mode.flag_control_manual_enabled
    wv_yaw_rate_max = par.auto_rate_max(3) * par.vtol_wv_yaw_rate_scale;
    rates_sp(3) = constrain(rates_sp(3), -wv_yaw_rate_max, wv_yaw_rate_max);
	%prevent integrator winding up in weathervane mode
	rates_int(3) = 0.0;
end

== matlab function pos_control2/attitude control/control_attitude_rates ==
  data: rates_sp input; rates_prev input; rates_int_prev input; thrust_sp input; attitude_vel input; att_control output; par parameter; rates output; rates_int output; def parameter; dt parameter
function [att_control,rates,rates_int] = control_attitude_rates(rates_sp, rates_prev,rates_int_prev ,thrust_sp, attitude_vel, par, def, dt)

rates_int = rates_int_prev;
%/* reset integral if disarmed */
%if (!_armed.armed || !_vehicle_status.is_rotary_wing) {
%rates_int = zero(1,3);
%}
%get the raw gyro data and correct for thermal errors

rates = zeros(3,1);

rates(1) = attitude_vel(1);
rates(2) = attitude_vel(2);
rates(3) = attitude_vel(3);
%rates(1) = (sensor_angular_vel(1) - sensor_offset(1)) * sensor_scale(1);
%rates(2) = (sensor_angular_vel(2) - sensor_offset(2)) * sensor_scale(2); 
%rates(3) = (sensor_angular_vel(3) - sensor_offset(3)) * sensor_scale(3); 

%rotate corrected measurements from sensor to body frame
%rates = par.board_rotation*rates;
%correct for in-run bias errors
%rates(1) = rates(1)-sensor_gyro_bias(1);
%rates(2) = rates(2)-sensor_gyro_bias(2);
%rates(3) = rates(3)-sensor_gyro_bias(3);

pid_p = pid_attenuations(par.tpa_breakpoint_p,par.tpa_rate_p,thrust_sp,def);
rates_p_scaled = [par.rate_p(1)*pid_p(1),par.rate_p(2)*pid_p(2),par.rate_p(3)*pid_p(3)]';

pid_d = pid_attenuations(par.tpa_breakpoint_d,par.tpa_rate_d,thrust_sp,def);
rates_d_scaled = [par.rate_d(1)*pid_d(1),par.rate_d(2)*pid_d(2),par.rate_d(3)*pid_d(3)]';

% angular rates error
rates_err = rates_sp - rates;

att_control = rates_p_scaled.*rates_err + rates_int + rates_d_scaled.*(rates_prev - rates)/dt + par.rate_ff.*rates_sp;

% update integral only if motors are providing enough thrust to be effective
if thrust_sp > def.MIN_TAKEOFF_THRUST
    for i = def.AXIS_INDEX_ROLL:def.AXIS_COUNT
        %Check for positive control saturation
        %todo
        %positive_saturation =((i == def.AXIS_INDEX_ROLL) && saturation_status.flags.roll_pos) ||((i == def.AXIS_INDEX_PITCH) && saturation_status.flags.pitch_pos) ||((i == def.AXIS_INDEX_YAW) && saturation_status.flags.yaw_pos);
        positive_saturation = 0;
		%Check for negative control saturation
        %negative_saturation =((i == def.AXIS_INDEX_ROLL) && saturation_status.flags.roll_neg) ||((i == def.AXIS_INDEX_PITCH) && saturation_status.flags.pitch_neg) ||((i == def.AXIS_INDEX_YAW) && saturation_status.flags.yaw_neg);
        negative_saturation = 0;
		%prevent further positive control saturation
        if (positive_saturation) 
            rates_err(i) = min(rates_err(i), 0.0);
        end

		%prevent further negative control saturation
        if (negative_saturation) 
            rates_err(i) = max(rates_err(i), 0.0);
        end
		
		%Perform the integration using a first order method and do not propaate the result if out of range or invalid
        rate_i = rates_int(i) + par.rate_i(i) * rates_err(i) * dt;
        
        if (rate_i > -par.rate_int_lim(i) && rate_i < par.rate_int_lim(i))
            rates_int(i) = rate_i;
        end
    end
end

%explicitly limit the integrator state */
for i = def.AXIS_INDEX_ROLL:def.AXIS_COUNT
    rates_int(i) = constrain(rates_int(i), -par.rate_int_lim(i), par.rate_int_lim(i));
end
